simulink model "TemporalEvent3"  (R2020b)
settings: Solver=VariableStepAuto  StartTime=0.0  StopTime=10.0  RelTol=1e-3
settings Model: Creator=apple  LastModifiedBy=apple

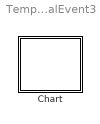
== system TemporalEvent3 ==
  Chart : Stateflow chart  TreatAsAtomicUnit=on

== stateflow chart TemporalEvent3/Chart ==
  state A
    en:fprintf("Entry A");
    du:fprintf("During A");
    ex:fprintf("Exit A");
    state A1
      en:fprintf("Entry A1");
      ex:fprintf("Exit A1");
    (default) -> A1
  state B
    en:fprintf("Entry B");
    du:fprintf("During B");
    ex:fprintf("Exit B");
  (default) -> A
  (junction 6) -> A1
  A -> B : after(3,E)
  A1 -> (junction 6)
  events: E local FUNCTION_CALL_EVENT
